simulink model "IEEE30_case"  (R2024b)
settings: Solver=FixedStepAuto  StartTime=0  StopTime=5  FixedStep=1e-7  RelTol=1e-3
values from neighbouring files (symbols this model uses):
  GFL_DFIG_7_C_bus = 0.08    [IEEE30_case_parameters.m]
  GFL_DFIG_7_D_mutual = 2.500000e+3    (= 2500)    [IEEE30_case_parameters.m]
  GFL_DFIG_7_f0 = 60    [IEEE30_case_parameters.m]
  GFL_DFIG_7_gPLLi = 3200    [IEEE30_case_parameters.m]
  GFL_DFIG_7_gPLLp = 650    [IEEE30_case_parameters.m]
  GFL_DFIG_7_H_WT = 0.4    [IEEE30_case_parameters.m]
  GFL_DFIG_7_Hg = 0.8    [IEEE30_case_parameters.m]
  GFL_DFIG_7_Igq_ref = 0    [IEEE30_case_parameters.m]
  GFL_DFIG_7_Ird_ref = 704.45696    [IEEE30_case_parameters.m]
  GFL_DFIG_7_KI_V = -300000    [IEEE30_case_parameters.m]
  GFL_DFIG_7_KP_V = -1000    [IEEE30_case_parameters.m]
  GFL_DFIG_7_Ksh = 1.254300e+4    (= 12543)    [IEEE30_case_parameters.m]
  GFL_DFIG_7_Lg = 0.000483    [IEEE30_case_parameters.m]
  GFL_DFIG_7_Lm_pu = 4    [IEEE30_case_parameters.m]
  GFL_DFIG_7_N = 100    [IEEE30_case_parameters.m]
  GFL_DFIG_7_p = 2    [IEEE30_case_parameters.m]
  GFL_DFIG_7_Pitch = 0    [IEEE30_case_parameters.m]
  GFL_DFIG_7_R = 44    [IEEE30_case_parameters.m]
  GFL_DFIG_7_Rg = 2.000000e-5    (= 2e-05)    [IEEE30_case_parameters.m]
  GFL_DFIG_7_rho = 1.225    [IEEE30_case_parameters.m]
  GFL_DFIG_7_rPLLi = 4500    [IEEE30_case_parameters.m]
  GFL_DFIG_7_rPLLp = 620    [IEEE30_case_parameters.m]
  GFL_DFIG_7_Rs_pu = 0.011    [IEEE30_case_parameters.m]
  GFL_DFIG_7_Sbase = 2.000000e+6    (= 2000000)    [IEEE30_case_parameters.m]
  GFL_DFIG_7_ugq_ref = 0    [IEEE30_case_parameters.m]
  GFL_DFIG_7_usd_ref = 0    [IEEE30_case_parameters.m]
  GFL_DFIG_7_Vbase = 690    [IEEE30_case_parameters.m]
  GFL_DFIG_7_Vdc_ref = 1200    [IEEE30_case_parameters.m]
  GFL_DFIG_7_wind = 12    [IEEE30_case_parameters.m]
  GFL_DFIG_7_wm_ref = 518.184209    [IEEE30_case_parameters.m]
  SG_D_13_D = 0.01056    [IEEE30_case_parameters.m]
  SG_D_13_EnableSaturation = 0    [IEEE30_case_parameters.m]
  SG_D_13_f0 = 60    [IEEE30_case_parameters.m]
  SG_D_13_H = 7.5    [IEEE30_case_parameters.m]
  SG_D_13_K_A = 20    [IEEE30_case_parameters.m]
  SG_D_13_K_E = 1.000000e+1    (= 10)    [IEEE30_case_parameters.m]
  SG_D_13_K_F = 2.363    [IEEE30_case_parameters.m]
  SG_D_13_K_s = 0.5    [IEEE30_case_parameters.m]
  SG_D_13_R_a = 0.001088    [IEEE30_case_parameters.m]
  SG_D_13_S_A = 1    [IEEE30_case_parameters.m]
  SG_D_13_S_B = 0.103    [IEEE30_case_parameters.m]
  SG_D_13_S_N = 10.659857    [IEEE30_case_parameters.m]
  SG_D_13_SpeedPara = 200    [IEEE30_case_parameters.m]
  SG_D_13_T_0 = 0.370163    [IEEE30_case_parameters.m]
  SG_D_13_T_1 = 0.3    [IEEE30_case_parameters.m]
  SG_D_13_T_2 = 0.05    [IEEE30_case_parameters.m]
  SG_D_13_T_3 = 0.02    [IEEE30_case_parameters.m]
  SG_D_13_T_4 = 0.005    [IEEE30_case_parameters.m]
  SG_D_13_T_A = 0.02    [IEEE30_case_parameters.m]
  SG_D_13_T_dd = 8.000000e+0    (= 8)    [IEEE30_case_parameters.m]
  SG_D_13_T_ddd = 0.04    [IEEE30_case_parameters.m]
  SG_D_13_T_E = 0.314    [IEEE30_case_parameters.m]
  SG_D_13_T_F = 0.35    [IEEE30_case_parameters.m]
  SG_D_13_T_qd = 0.8    [IEEE30_case_parameters.m]
  SG_D_13_T_qdd = 0.02    [IEEE30_case_parameters.m]
  SG_D_13_T_speed = 0.1    [IEEE30_case_parameters.m]
  SG_D_13_T_w = 0.5    [IEEE30_case_parameters.m]
  SG_D_13_V_ref = 1.696619    [IEEE30_case_parameters.m]
  SG_D_13_w_ref = 376.991118    [IEEE30_case_parameters.m]
  SG_D_13_x_d = 1.9    [IEEE30_case_parameters.m]
  SG_D_13_x_dd = 0.302    [IEEE30_case_parameters.m]
  SG_D_13_x_ddd = 0.204    [IEEE30_case_parameters.m]
  SG_D_13_x_l = 0.05    [IEEE30_case_parameters.m]
  SG_D_13_x_q = 1.3    [IEEE30_case_parameters.m]
  SG_D_13_x_qd = 0.5    [IEEE30_case_parameters.m]
  SG_D_13_x_qdd = 0.3    [IEEE30_case_parameters.m]
  SG_D_1_D = 0.01056    [IEEE30_case_parameters.m]
  SG_D_1_EnableSaturation = 0    [IEEE30_case_parameters.m]
  SG_D_1_f0 = 60    [IEEE30_case_parameters.m]
  SG_D_1_H = 7.5    [IEEE30_case_parameters.m]
  SG_D_1_K_A = 20    [IEEE30_case_parameters.m]
  SG_D_1_K_E = 1.000000e+1    (= 10)    [IEEE30_case_parameters.m]
  SG_D_1_K_F = 2.363    [IEEE30_case_parameters.m]
  SG_D_1_K_s = 0.5    [IEEE30_case_parameters.m]
  SG_D_1_R_a = 0.001088    [IEEE30_case_parameters.m]
  SG_D_1_S_A = 1    [IEEE30_case_parameters.m]
  SG_D_1_S_B = 0.103    [IEEE30_case_parameters.m]
  SG_D_1_S_N = 10.659857    [IEEE30_case_parameters.m]
  SG_D_1_SpeedPara = 200    [IEEE30_case_parameters.m]
  SG_D_1_T_0 = 0.259812    [IEEE30_case_parameters.m]
  SG_D_1_T_1 = 0.3    [IEEE30_case_parameters.m]
  SG_D_1_T_2 = 0.05    [IEEE30_case_parameters.m]
  SG_D_1_T_3 = 0.02    [IEEE30_case_parameters.m]
  SG_D_1_T_4 = 0.005    [IEEE30_case_parameters.m]
  SG_D_1_T_A = 0.02    [IEEE30_case_parameters.m]
  SG_D_1_T_dd = 8.000000e+0    (= 8)    [IEEE30_case_parameters.m]
  SG_D_1_T_ddd = 0.04    [IEEE30_case_parameters.m]
  SG_D_1_T_E = 0.314    [IEEE30_case_parameters.m]
  SG_D_1_T_F = 0.35    [IEEE30_case_parameters.m]
  SG_D_1_T_qd = 0.8    [IEEE30_case_parameters.m]
  SG_D_1_T_qdd = 0.02    [IEEE30_case_parameters.m]
  SG_D_1_T_speed = 0.1    [IEEE30_case_parameters.m]
  SG_D_1_T_w = 0.5    [IEEE30_case_parameters.m]
  SG_D_1_V_ref = 1.544107    [IEEE30_case_parameters.m]
  SG_D_1_w_ref = 376.991118    [IEEE30_case_parameters.m]
  SG_D_1_x_d = 1.9    [IEEE30_case_parameters.m]
  SG_D_1_x_dd = 0.302    [IEEE30_case_parameters.m]
  SG_D_1_x_ddd = 0.204    [IEEE30_case_parameters.m]
  SG_D_1_x_l = 0.05    [IEEE30_case_parameters.m]
  SG_D_1_x_q = 1.3    [IEEE30_case_parameters.m]
  SG_D_1_x_qd = 0.5    [IEEE30_case_parameters.m]
  SG_D_1_x_qdd = 0.3    [IEEE30_case_parameters.m]
  SG_D_22_D = 0.01056    [IEEE30_case_parameters.m]
  SG_D_22_EnableSaturation = 0    [IEEE30_case_parameters.m]
  SG_D_22_f0 = 60    [IEEE30_case_parameters.m]
  SG_D_22_H = 7.5    [IEEE30_case_parameters.m]
  SG_D_22_K_A = 20    [IEEE30_case_parameters.m]
  SG_D_22_K_E = 1.000000e+1    (= 10)    [IEEE30_case_parameters.m]
  SG_D_22_K_F = 2.363    [IEEE30_case_parameters.m]
  SG_D_22_K_s = 0.5    [IEEE30_case_parameters.m]
  SG_D_22_R_a = 0.001088    [IEEE30_case_parameters.m]
  SG_D_22_S_A = 1    [IEEE30_case_parameters.m]
  SG_D_22_S_B = 0.103    [IEEE30_case_parameters.m]
  SG_D_22_S_N = 10.659857    [IEEE30_case_parameters.m]
  SG_D_22_SpeedPara = 200    [IEEE30_case_parameters.m]
  SG_D_22_T_0 = 0.216121    [IEEE30_case_parameters.m]
  SG_D_22_T_1 = 0.3    [IEEE30_case_parameters.m]
  SG_D_22_T_2 = 0.05    [IEEE30_case_parameters.m]
  SG_D_22_T_3 = 0.02    [IEEE30_case_parameters.m]
  SG_D_22_T_4 = 0.005    [IEEE30_case_parameters.m]
  ... (+126 more)
(part 11 of 27)

== system IEEE30_case/AC_1/iq_bus_12_block ==
  note: iq_bus_12 in IEEE30_case
      | $\mathrm{iq}_{\mathrm{line},4,12}-\mathrm{iq}_{\mathrm{load},12}-\mathrm{iq}_{\mathrm{line},12,13}-\mathrm{iq}_{\mathrm{line},12,14}-\mathrm{iq}_{\mathrm{line},12,15}-\mathrm{iq}_{\mathrm{line},12,16}$
      | Automatically generated on 2025-11-01 18:42:55 .
  State_iq_load_12_bc973 : Inport
  State_iq_line_4_12_d3882 : Inport  Port=2
  State_iq_line_12_13_64934 : Inport  Port=3
  State_iq_line_12_14_05407 : Inport  Port=4
  State_iq_line_12_15_032f0 : Inport  Port=5
  State_iq_line_12_16_bc787 : Inport  Port=6
  Add_841f8 : Sum
  Constant_-1_4865d : Constant  Value=-1
  Product_64089 : Product
  Subtract_44be1 : Sum  Inputs=+-
  Subtract_8e198 : Sum  Inputs=+-
  Subtract_b2fb8 : Sum  Inputs=+-
  Subtract_d73aa : Sum  Inputs=+-
  Blockout_iq_bus_12_94dfd : Outport
  wires:
  State_iq_line_4_12_d3882/1 -> Add_841f8/2
  Constant_-1_4865d/1 -> Product_64089/1
  Product_64089/1 -> Add_841f8/1
  State_iq_load_12_bc973/1 -> Product_64089/2
  State_iq_line_12_14_05407/1 -> Subtract_44be1/2
  Subtract_8e198/1 -> Subtract_d73aa/1
  Add_841f8/1 -> Subtract_b2fb8/1
  Subtract_b2fb8/1 -> Subtract_44be1/1
  State_iq_line_12_13_64934/1 -> Subtract_b2fb8/2
  Subtract_44be1/1 -> Subtract_8e198/1
  State_iq_line_12_15_032f0/1 -> Subtract_8e198/2
  State_iq_line_12_16_bc787/1 -> Subtract_d73aa/2
  Subtract_d73aa/1 -> Blockout_iq_bus_12_94dfd/1

== system IEEE30_case/AC_1/iq_bus_13_block ==
  note: iq_bus_13 in IEEE30_case
      | $\mathrm{iq}_{\mathrm{SG},D,13}+\mathrm{iq}_{\mathrm{line},12,13}$
      | Automatically generated on 2025-11-01 18:42:58 .
  Input_iq_SG_D_13_41b6f : Inport
  State_iq_line_12_13_2e588 : Inport  Port=2
  Add_10a27 : Sum
  Blockout_iq_bus_13_72f64 : Outport
  wires:
  Input_iq_SG_D_13_41b6f/1 -> Add_10a27/1
  State_iq_line_12_13_2e588/1 -> Add_10a27/2
  Add_10a27/1 -> Blockout_iq_bus_13_72f64/1

== system IEEE30_case/AC_1/iq_bus_14_block ==
  note: iq_bus_14 in IEEE30_case
      | $\mathrm{iq}_{\mathrm{line},12,14}-\mathrm{iq}_{\mathrm{load},14}-\mathrm{iq}_{\mathrm{line},14,15}$
      | Automatically generated on 2025-11-01 18:42:59 .
  State_iq_load_14_72e79 : Inport
  State_iq_line_12_14_c9961 : Inport  Port=2
  State_iq_line_14_15_62994 : Inport  Port=3
  Add_1995a : Sum
  Constant_-1_aea63 : Constant  Value=-1
  Product_4bd77 : Product
  Subtract_3c8e1 : Sum  Inputs=+-
  Blockout_iq_bus_14_40877 : Outport
  wires:
  State_iq_line_14_15_62994/1 -> Subtract_3c8e1/2
  State_iq_line_12_14_c9961/1 -> Add_1995a/2
  Product_4bd77/1 -> Add_1995a/1
  Constant_-1_aea63/1 -> Product_4bd77/1
  State_iq_load_14_72e79/1 -> Product_4bd77/2
  Add_1995a/1 -> Subtract_3c8e1/1
  Subtract_3c8e1/1 -> Blockout_iq_bus_14_40877/1

== system IEEE30_case/AC_1/iq_bus_15_block ==
  note: iq_bus_15 in IEEE30_case
      | $\mathrm{iq}_{\mathrm{line},12,15}-\mathrm{iq}_{\mathrm{load},15}+\mathrm{iq}_{\mathrm{line},14,15}-\mathrm{iq}_{\mathrm{line},15,18}-\mathrm{iq}_{\mathrm{line},15,23}$
      | Automatically generated on 2025-11-01 18:43:01 .
  State_iq_load_15_d1891 : Inport
  State_iq_line_12_15_d11d7 : Inport  Port=2
  State_iq_line_14_15_cd3f2 : Inport  Port=3
  State_iq_line_15_18_a2738 : Inport  Port=4
  State_iq_line_15_23_dd72a : Inport  Port=5
  Add_86658 : Sum
  Add_f7d0d : Sum
  Constant_-1_2c9e4 : Constant  Value=-1
  Product_847ef : Product
  Subtract_29d9d : Sum  Inputs=+-
  Subtract_4ac4f : Sum  Inputs=+-
  Blockout_iq_bus_15_ccbd2 : Outport
  wires:
  State_iq_line_14_15_cd3f2/1 -> Add_f7d0d/2
  Subtract_4ac4f/1 -> Subtract_29d9d/1
  State_iq_line_12_15_d11d7/1 -> Add_86658/2
  Constant_-1_2c9e4/1 -> Product_847ef/1
  Product_847ef/1 -> Add_86658/1
  State_iq_load_15_d1891/1 -> Product_847ef/2
  State_iq_line_15_18_a2738/1 -> Subtract_4ac4f/2
  Add_86658/1 -> Add_f7d0d/1
  Add_f7d0d/1 -> Subtract_4ac4f/1
  State_iq_line_15_23_dd72a/1 -> Subtract_29d9d/2
  Subtract_29d9d/1 -> Blockout_iq_bus_15_ccbd2/1

== system IEEE30_case/AC_1/iq_bus_16_block ==
  note: iq_bus_16 in IEEE30_case
      | $\mathrm{iq}_{\mathrm{line},12,16}-\mathrm{iq}_{\mathrm{load},16}-\mathrm{iq}_{\mathrm{line},16,17}$
      | Automatically generated on 2025-11-01 18:43:03 .
  State_iq_load_16_aacc5 : Inport
  State_iq_line_12_16_8d22f : Inport  Port=2
  State_iq_line_16_17_2d89b : Inport  Port=3
  Add_8c6a6 : Sum
  Constant_-1_7911e : Constant  Value=-1
  Product_fbab2 : Product
  Subtract_cf134 : Sum  Inputs=+-
  Blockout_iq_bus_16_0845b : Outport
  wires:
  Product_fbab2/1 -> Add_8c6a6/1
  Constant_-1_7911e/1 -> Product_fbab2/1
  State_iq_load_16_aacc5/1 -> Product_fbab2/2
  State_iq_line_16_17_2d89b/1 -> Subtract_cf134/2
  Add_8c6a6/1 -> Subtract_cf134/1
  State_iq_line_12_16_8d22f/1 -> Add_8c6a6/2
  Subtract_cf134/1 -> Blockout_iq_bus_16_0845b/1

== system IEEE30_case/AC_1/iq_bus_17_block ==
  note: iq_bus_17 in IEEE30_case
      | $\mathrm{iq}_{\mathrm{line},10,17}-\mathrm{iq}_{\mathrm{load},17}+\mathrm{iq}_{\mathrm{line},16,17}$
      | Automatically generated on 2025-11-01 18:43:05 .
  State_iq_load_17_c996c : Inport
  State_iq_line_10_17_8adde : Inport  Port=2
  State_iq_line_16_17_d8ac8 : Inport  Port=3
  Add_26423 : Sum
  Add_c9bbe : Sum
  Constant_-1_1ae42 : Constant  Value=-1
  Product_876e2 : Product
  Blockout_iq_bus_17_f1a33 : Outport
  wires:
  Add_c9bbe/1 -> Blockout_iq_bus_17_f1a33/1
  Constant_-1_1ae42/1 -> Product_876e2/1
  State_iq_load_17_c996c/1 -> Product_876e2/2
  Product_876e2/1 -> Add_26423/1
  State_iq_line_16_17_d8ac8/1 -> Add_c9bbe/2
  Add_26423/1 -> Add_c9bbe/1
  State_iq_line_10_17_8adde/1 -> Add_26423/2

== system IEEE30_case/AC_1/iq_bus_18_block ==
  note: iq_bus_18 in IEEE30_case
      | $\mathrm{iq}_{\mathrm{line},15,18}-\mathrm{iq}_{\mathrm{load},18}-\mathrm{iq}_{\mathrm{line},18,19}$
      | Automatically generated on 2025-11-01 18:43:06 .
  State_iq_load_18_b73eb : Inport
  State_iq_line_15_18_3f1e8 : Inport  Port=2
  State_iq_line_18_19_1de76 : Inport  Port=3
  Add_094f5 : Sum
  Constant_-1_fe84d : Constant  Value=-1
  Product_a729b : Product
  Subtract_f2aa7 : Sum  Inputs=+-
  Blockout_iq_bus_18_b4916 : Outport
  wires:
  Subtract_f2aa7/1 -> Blockout_iq_bus_18_b4916/1
  Product_a729b/1 -> Add_094f5/1
  Constant_-1_fe84d/1 -> Product_a729b/1
  State_iq_line_15_18_3f1e8/1 -> Add_094f5/2
  State_iq_load_18_b73eb/1 -> Product_a729b/2
  Add_094f5/1 -> Subtract_f2aa7/1
  State_iq_line_18_19_1de76/1 -> Subtract_f2aa7/2

== system IEEE30_case/AC_1/iq_bus_19_block ==
  note: iq_bus_19 in IEEE30_case
      | $\mathrm{iq}_{\mathrm{line},18,19}-\mathrm{iq}_{\mathrm{load},19}-\mathrm{iq}_{\mathrm{line},19,20}$
      | Automatically generated on 2025-11-01 18:43:08 .
  State_iq_load_19_c9423 : Inport
  State_iq_line_18_19_b0a61 : Inport  Port=2
  State_iq_line_19_20_3626a : Inport  Port=3
  Add_da601 : Sum
  Constant_-1_3887f : Constant  Value=-1
  Product_3a158 : Product
  Subtract_a6f15 : Sum  Inputs=+-
  Blockout_iq_bus_19_07988 : Outport
  wires:
  State_iq_line_18_19_b0a61/1 -> Add_da601/2
  Product_3a158/1 -> Add_da601/1
  Constant_-1_3887f/1 -> Product_3a158/1
  State_iq_load_19_c9423/1 -> Product_3a158/2
  Add_da601/1 -> Subtract_a6f15/1
  State_iq_line_19_20_3626a/1 -> Subtract_a6f15/2
  Subtract_a6f15/1 -> Blockout_iq_bus_19_07988/1

== system IEEE30_case/AC_1/iq_bus_1_block ==
  note: iq_bus_1 in IEEE30_case
      | $\mathrm{iq}_{\mathrm{SG},D,1}-\mathrm{iq}_{\mathrm{line},1,2}-\mathrm{iq}_{\mathrm{line},1,3}$
      | Automatically generated on 2025-11-01 18:42:34 .
  Input_iq_SG_D_1_636be : Inport
  State_iq_line_1_2_426df : Inport  Port=2
  State_iq_line_1_3_a1a02 : Inport  Port=3
  Subtract_baca8 : Sum  Inputs=+-
  Subtract_effd5 : Sum  Inputs=+-
  Blockout_iq_bus_1_c22d8 : Outport
  wires:
  Subtract_baca8/1 -> Blockout_iq_bus_1_c22d8/1
  Input_iq_SG_D_1_636be/1 -> Subtract_effd5/1
  State_iq_line_1_3_a1a02/1 -> Subtract_baca8/2
  State_iq_line_1_2_426df/1 -> Subtract_effd5/2
  Subtract_effd5/1 -> Subtract_baca8/1

== system IEEE30_case/AC_1/iq_bus_20_block ==
  note: iq_bus_20 in IEEE30_case
      | $\mathrm{iq}_{\mathrm{line},10,20}-\mathrm{iq}_{\mathrm{load},20}+\mathrm{iq}_{\mathrm{line},19,20}$
      | Automatically generated on 2025-11-01 18:43:10 .
  State_iq_load_20_1f6b7 : Inport
  State_iq_line_10_20_d570b : Inport  Port=2
  State_iq_line_19_20_435ec : Inport  Port=3
  Add_2092f : Sum
  Add_2fcde : Sum
  Constant_-1_9ffd8 : Constant  Value=-1
  Product_27044 : Product
  Blockout_iq_bus_20_faa95 : Outport
  wires:
  Add_2092f/1 -> Add_2fcde/1
  Product_27044/1 -> Add_2092f/1
  Constant_-1_9ffd8/1 -> Product_27044/1
  State_iq_load_20_1f6b7/1 -> Product_27044/2
  Add_2fcde/1 -> Blockout_iq_bus_20_faa95/1
  State_iq_line_19_20_435ec/1 -> Add_2fcde/2
  State_iq_line_10_20_d570b/1 -> Add_2092f/2

== system IEEE30_case/AC_1/iq_bus_21_block ==
  note: iq_bus_21 in IEEE30_case
      | $\mathrm{iq}_{\mathrm{line},10,21}-\mathrm{iq}_{\mathrm{load},21}-\mathrm{iq}_{\mathrm{line},21,22}$
      | Automatically generated on 2025-11-01 18:43:11 .
  State_iq_load_21_44508 : Inport
  State_iq_line_10_21_86c36 : Inport  Port=2
  State_iq_line_21_22_832b6 : Inport  Port=3
  Add_22f1e : Sum
  Constant_-1_58c82 : Constant  Value=-1
  Product_c246b : Product
  Subtract_625b5 : Sum  Inputs=+-
  Blockout_iq_bus_21_51471 : Outport
  wires:
  State_iq_line_21_22_832b6/1 -> Subtract_625b5/2
  State_iq_line_10_21_86c36/1 -> Add_22f1e/2
  Constant_-1_58c82/1 -> Product_c246b/1
  State_iq_load_21_44508/1 -> Product_c246b/2
  Product_c246b/1 -> Add_22f1e/1
  Add_22f1e/1 -> Subtract_625b5/1
  Subtract_625b5/1 -> Blockout_iq_bus_21_51471/1

== system IEEE30_case/AC_1/iq_bus_22_block ==
  note: iq_bus_22 in IEEE30_case
      | $\mathrm{iq}_{\mathrm{SG},D,22}+\mathrm{iq}_{\mathrm{line},10,22}+\mathrm{iq}_{\mathrm{line},21,22}-\mathrm{iq}_{\mathrm{line},22,24}$
      | Automatically generated on 2025-11-01 18:43:14 .
  Input_iq_SG_D_22_7afaf : Inport
  State_iq_line_10_22_172f8 : Inport  Port=2
  State_iq_line_21_22_a7d32 : Inport  Port=3
  State_iq_line_22_24_573df : Inport  Port=4
  Add_60857 : Sum
  Add_ff722 : Sum
  Subtract_94456 : Sum  Inputs=+-
  Blockout_iq_bus_22_6516e : Outport
  wires:
  Subtract_94456/1 -> Blockout_iq_bus_22_6516e/1
  Add_ff722/1 -> Add_60857/1
  Input_iq_SG_D_22_7afaf/1 -> Add_ff722/1
  State_iq_line_10_22_172f8/1 -> Add_ff722/2
  Add_60857/1 -> Subtract_94456/1
  State_iq_line_21_22_a7d32/1 -> Add_60857/2
  State_iq_line_22_24_573df/1 -> Subtract_94456/2

== system IEEE30_case/AC_1/iq_bus_23_block ==
  note: iq_bus_23 in IEEE30_case
      | $\mathrm{iq}_{\mathrm{SG},D,23}-\mathrm{iq}_{\mathrm{load},23}+\mathrm{iq}_{\mathrm{line},15,23}-\mathrm{iq}_{\mathrm{line},23,24}$
      | Automatically generated on 2025-11-01 18:43:17 .
  Input_iq_SG_D_23_15e34 : Inport
  State_iq_load_23_12e45 : Inport  Port=2
  State_iq_line_15_23_fc0a9 : Inport  Port=3
  State_iq_line_23_24_17ece : Inport  Port=4
  Add_e4154 : Sum
  Subtract_5918e : Sum  Inputs=+-
  Subtract_8e4ad : Sum  Inputs=+-
  Blockout_iq_bus_23_896ad : Outport
  wires:
  Subtract_8e4ad/1 -> Add_e4154/1
  Input_iq_SG_D_23_15e34/1 -> Subtract_8e4ad/1
  State_iq_load_23_12e45/1 -> Subtract_8e4ad/2
  State_iq_line_23_24_17ece/1 -> Subtract_5918e/2
  Add_e4154/1 -> Subtract_5918e/1
  State_iq_line_15_23_fc0a9/1 -> Add_e4154/2
  Subtract_5918e/1 -> Blockout_iq_bus_23_896ad/1

== system IEEE30_case/AC_1/iq_bus_24_block ==
  note: iq_bus_24 in IEEE30_case
      | $\mathrm{iq}_{\mathrm{line},22,24}-\mathrm{iq}_{\mathrm{load},24}+\mathrm{iq}_{\mathrm{line},23,24}-\mathrm{iq}_{\mathrm{line},24,25}$
      | Automatically generated on 2025-11-01 18:43:19 .
  State_iq_load_24_fdcb6 : Inport
  State_iq_line_22_24_76281 : Inport  Port=2
  State_iq_line_23_24_946d1 : Inport  Port=3
  State_iq_line_24_25_99c0f : Inport  Port=4
  Add_5c6aa : Sum
  Add_67e83 : Sum
  Constant_-1_ac1a7 : Constant  Value=-1
  Product_7a246 : Product
  Subtract_26d4f : Sum  Inputs=+-
  Blockout_iq_bus_24_a8f54 : Outport
  wires:
  Constant_-1_ac1a7/1 -> Product_7a246/1
  Product_7a246/1 -> Add_5c6aa/1
  Add_67e83/1 -> Subtract_26d4f/1
  Add_5c6aa/1 -> Add_67e83/1
  State_iq_load_24_fdcb6/1 -> Product_7a246/2
  State_iq_line_22_24_76281/1 -> Add_5c6aa/2
  State_iq_line_24_25_99c0f/1 -> Subtract_26d4f/2
  State_iq_line_23_24_946d1/1 -> Add_67e83/2
  Subtract_26d4f/1 -> Blockout_iq_bus_24_a8f54/1

== system IEEE30_case/AC_1/iq_bus_25_block ==
  note: iq_bus_25 in IEEE30_case
      | $\mathrm{iq}_{\mathrm{line},24,25}-\mathrm{iq}_{\mathrm{line},25,26}-\mathrm{iq}_{\mathrm{line},25,27}$
      | Automatically generated on 2025-11-01 18:43:21 .
  State_iq_line_24_25_0047e : Inport
  State_iq_line_25_26_b28ea : Inport  Port=2
  State_iq_line_25_27_6cee1 : Inport  Port=3
  Subtract_623d2 : Sum  Inputs=+-
  Subtract_b39cd : Sum  Inputs=+-
  Blockout_iq_bus_25_a2b76 : Outport
  wires:
  Subtract_b39cd/1 -> Blockout_iq_bus_25_a2b76/1
  State_iq_line_24_25_0047e/1 -> Subtract_623d2/1
  State_iq_line_25_26_b28ea/1 -> Subtract_623d2/2
  State_iq_line_25_27_6cee1/1 -> Subtract_b39cd/2
  Subtract_623d2/1 -> Subtract_b39cd/1

== system IEEE30_case/AC_1/iq_bus_26_block ==
  note: iq_bus_26 in IEEE30_case
      | $\mathrm{iq}_{\mathrm{line},25,26}-\mathrm{iq}_{\mathrm{load},26}$
      | Automatically generated on 2025-11-01 18:43:22 .
  State_iq_load_26_ac2a5 : Inport
  State_iq_line_25_26_3a876 : Inport  Port=2
  Add_463e9 : Sum
  Constant_-1_82269 : Constant  Value=-1
  Product_c91b9 : Product
  Blockout_iq_bus_26_d1a08 : Outport
  wires:
  Constant_-1_82269/1 -> Product_c91b9/1
  State_iq_line_25_26_3a876/1 -> Add_463e9/2
  Product_c91b9/1 -> Add_463e9/1
  State_iq_load_26_ac2a5/1 -> Product_c91b9/2
  Add_463e9/1 -> Blockout_iq_bus_26_d1a08/1

== system IEEE30_case/AC_1/iq_bus_27_block ==
  note: iq_bus_27 in IEEE30_case
      | $\mathrm{iq}_{\mathrm{SG},D,27}+\mathrm{iq}_{\mathrm{line},25,27}-\mathrm{iq}_{\mathrm{line},27,29}-\mathrm{iq}_{\mathrm{line},27,30}+\mathrm{iq}_{\mathrm{line},28,27}$
      | Automatically generated on 2025-11-01 18:43:25 .
  Input_iq_SG_D_27_5f248 : Inport
  State_iq_line_25_27_786f4 : Inport  Port=2
  State_iq_line_27_29_e7090 : Inport  Port=3
  State_iq_line_27_30_e8aeb : Inport  Port=4
  State_iq_line_28_27_c8698 : Inport  Port=5
  Add_88ff4 : Sum
  Add_a91b2 : Sum
  Subtract_49574 : Sum  Inputs=+-
  Subtract_f659e : Sum  Inputs=+-
  Blockout_iq_bus_27_6c5f3 : Outport
  wires:
  Subtract_f659e/1 -> Add_88ff4/1
  Input_iq_SG_D_27_5f248/1 -> Add_a91b2/1
  Add_a91b2/1 -> Subtract_49574/1
  Subtract_49574/1 -> Subtract_f659e/1
  State_iq_line_25_27_786f4/1 -> Add_a91b2/2
  State_iq_line_27_29_e7090/1 -> Subtract_49574/2
  State_iq_line_28_27_c8698/1 -> Add_88ff4/2
  State_iq_line_27_30_e8aeb/1 -> Subtract_f659e/2
  Add_88ff4/1 -> Blockout_iq_bus_27_6c5f3/1

== system IEEE30_case/AC_1/iq_bus_28_block ==
  note: iq_bus_28 in IEEE30_case
      | $\mathrm{iq}_{\mathrm{line},6,28}+\mathrm{iq}_{\mathrm{line},8,28}-\mathrm{iq}_{\mathrm{line},28,27}$
      | Automatically generated on 2025-11-01 18:43:27 .
  State_iq_line_6_28_9fc56 : Inport
  State_iq_line_8_28_5df2a : Inport  Port=2
  State_iq_line_28_27_5cab2 : Inport  Port=3
  Add_68cf3 : Sum
  Subtract_c2c34 : Sum  Inputs=+-
  Blockout_iq_bus_28_fc1de : Outport
  wires:
  Subtract_c2c34/1 -> Blockout_iq_bus_28_fc1de/1
  State_iq_line_6_28_9fc56/1 -> Add_68cf3/1
  State_iq_line_8_28_5df2a/1 -> Add_68cf3/2
  Add_68cf3/1 -> Subtract_c2c34/1
  State_iq_line_28_27_5cab2/1 -> Subtract_c2c34/2

== system IEEE30_case/AC_1/iq_bus_29_block ==
  note: iq_bus_29 in IEEE30_case
      | $\mathrm{iq}_{\mathrm{line},27,29}-\mathrm{iq}_{\mathrm{load},29}-\mathrm{iq}_{\mathrm{line},29,30}$
      | Automatically generated on 2025-11-01 18:43:28 .
  State_iq_load_29_82b4e : Inport
  State_iq_line_27_29_eb40a : Inport  Port=2
  State_iq_line_29_30_aaab3 : Inport  Port=3
  Add_05210 : Sum
  Constant_-1_1f122 : Constant  Value=-1
  Product_41592 : Product
  Subtract_864dd : Sum  Inputs=+-
  Blockout_iq_bus_29_54fcd : Outport
  wires:
  Subtract_864dd/1 -> Blockout_iq_bus_29_54fcd/1
  Product_41592/1 -> Add_05210/1
  Constant_-1_1f122/1 -> Product_41592/1
  State_iq_load_29_82b4e/1 -> Product_41592/2
  State_iq_line_27_29_eb40a/1 -> Add_05210/2
  Add_05210/1 -> Subtract_864dd/1
  State_iq_line_29_30_aaab3/1 -> Subtract_864dd/2

== system IEEE30_case/AC_1/iq_bus_2_block ==
  note: iq_bus_2 in IEEE30_case
      | $\mathrm{iq}_{\mathrm{SG},D,2}-\mathrm{iq}_{\mathrm{load},2}+\mathrm{iq}_{\mathrm{line},1,2}-\mathrm{iq}_{\mathrm{line},2,4}-\mathrm{iq}_{\mathrm{line},2,5}-\mathrm{iq}_{\mathrm{line},2,6}$
      | Automatically generated on 2025-11-01 18:42:36 .
  Input_iq_SG_D_2_3deae : Inport
  State_iq_load_2_becb6 : Inport  Port=2
  State_iq_line_1_2_22297 : Inport  Port=3
  State_iq_line_2_4_c1409 : Inport  Port=4
  State_iq_line_2_5_9d19f : Inport  Port=5
  State_iq_line_2_6_42b8c : Inport  Port=6
  Add_32615 : Sum
  Subtract_354fb : Sum  Inputs=+-
  Subtract_3c630 : Sum  Inputs=+-
  Subtract_b2643 : Sum  Inputs=+-
  Subtract_bac10 : Sum  Inputs=+-
  Blockout_iq_bus_2_bb89e : Outport
  wires:
  State_iq_line_1_2_22297/1 -> Add_32615/2
  Input_iq_SG_D_2_3deae/1 -> Subtract_b2643/1
  Subtract_b2643/1 -> Add_32615/1
  State_iq_load_2_becb6/1 -> Subtract_b2643/2
  State_iq_line_2_5_9d19f/1 -> Subtract_354fb/2
  State_iq_line_2_4_c1409/1 -> Subtract_bac10/2
  Add_32615/1 -> Subtract_bac10/1
  Subtract_bac10/1 -> Subtract_354fb/1
  Subtract_354fb/1 -> Subtract_3c630/1
  State_iq_line_2_6_42b8c/1 -> Subtract_3c630/2
  Subtract_3c630/1 -> Blockout_iq_bus_2_bb89e/1

== system IEEE30_case/AC_1/iq_bus_30_block ==
  note: iq_bus_30 in IEEE30_case
      | $\mathrm{iq}_{\mathrm{line},27,30}-\mathrm{iq}_{\mathrm{load},30}+\mathrm{iq}_{\mathrm{line},29,30}$
      | Automatically generated on 2025-11-01 18:43:30 .
  State_iq_load_30_e4c4c : Inport
  State_iq_line_27_30_c3531 : Inport  Port=2
  State_iq_line_29_30_a165e : Inport  Port=3
  Add_2918f : Sum
  Add_b8be3 : Sum
  Constant_-1_8c75b : Constant  Value=-1
  Product_583d8 : Product
  Blockout_iq_bus_30_f5578 : Outport
  wires:
  State_iq_line_29_30_a165e/1 -> Add_b8be3/2
  State_iq_line_27_30_c3531/1 -> Add_2918f/2
  Product_583d8/1 -> Add_2918f/1
  Constant_-1_8c75b/1 -> Product_583d8/1
  State_iq_load_30_e4c4c/1 -> Product_583d8/2
  Add_2918f/1 -> Add_b8be3/1
  Add_b8be3/1 -> Blockout_iq_bus_30_f5578/1

== system IEEE30_case/AC_1/iq_bus_3_block ==
  note: iq_bus_3 in IEEE30_case
      | $\mathrm{iq}_{\mathrm{line},1,3}-\mathrm{iq}_{\mathrm{load},3}-\mathrm{iq}_{\mathrm{line},3,4}$
      | Automatically generated on 2025-11-01 18:42:38 .
  State_iq_load_3_98680 : Inport
  State_iq_line_1_3_704f9 : Inport  Port=2
  State_iq_line_3_4_e67cb : Inport  Port=3
  Add_9cf2e : Sum
  Constant_-1_14019 : Constant  Value=-1
  Product_a35fa : Product
  Subtract_a74b4 : Sum  Inputs=+-
  Blockout_iq_bus_3_0811d : Outport
  wires:
  Product_a35fa/1 -> Add_9cf2e/1
  Constant_-1_14019/1 -> Product_a35fa/1
  State_iq_load_3_98680/1 -> Product_a35fa/2
  Add_9cf2e/1 -> Subtract_a74b4/1
  State_iq_line_1_3_704f9/1 -> Add_9cf2e/2
  State_iq_line_3_4_e67cb/1 -> Subtract_a74b4/2
  Subtract_a74b4/1 -> Blockout_iq_bus_3_0811d/1

== system IEEE30_case/AC_1/iq_bus_4_block ==
  note: iq_bus_4 in IEEE30_case
      | $\mathrm{iq}_{\mathrm{line},2,4}-\mathrm{iq}_{\mathrm{load},4}+\mathrm{iq}_{\mathrm{line},3,4}-\mathrm{iq}_{\mathrm{line},4,6}-\mathrm{iq}_{\mathrm{line},4,12}$
      | Automatically generated on 2025-11-01 18:42:40 .
  State_iq_load_4_0a7a4 : Inport
  State_iq_line_2_4_37eb2 : Inport  Port=2
  State_iq_line_3_4_5b109 : Inport  Port=3
  State_iq_line_4_6_d2f2a : Inport  Port=4
  State_iq_line_4_12_8cce3 : Inport  Port=5
  Add_5198b : Sum
  Add_8557f : Sum
  Constant_-1_cc943 : Constant  Value=-1
  Product_6109f : Product
  Subtract_850d4 : Sum  Inputs=+-
  Subtract_9ef8a : Sum  Inputs=+-
  Blockout_iq_bus_4_c8ef1 : Outport
  wires:
  Constant_-1_cc943/1 -> Product_6109f/1
  Product_6109f/1 -> Add_8557f/1
  State_iq_load_4_0a7a4/1 -> Product_6109f/2
  State_iq_line_2_4_37eb2/1 -> Add_8557f/2
  Add_8557f/1 -> Add_5198b/1
  State_iq_line_4_6_d2f2a/1 -> Subtract_850d4/2
  State_iq_line_3_4_5b109/1 -> Add_5198b/2
  Add_5198b/1 -> Subtract_850d4/1
  Subtract_850d4/1 -> Subtract_9ef8a/1
  State_iq_line_4_12_8cce3/1 -> Subtract_9ef8a/2
  Subtract_9ef8a/1 -> Blockout_iq_bus_4_c8ef1/1

== system IEEE30_case/AC_1/iq_bus_5_block ==
  note: iq_bus_5 in IEEE30_case
      | $\mathrm{iq}_{\mathrm{line},2,5}-\mathrm{iq}_{\mathrm{line},5,7}$
      | Automatically generated on 2025-11-01 18:42:41 .
  State_iq_line_2_5_98d2b : Inport
  State_iq_line_5_7_0b183 : Inport  Port=2
  Subtract_b6711 : Sum  Inputs=+-
  Blockout_iq_bus_5_aa6f8 : Outport
  wires:
  State_iq_line_5_7_0b183/1 -> Subtract_b6711/2
  State_iq_line_2_5_98d2b/1 -> Subtract_b6711/1
  Subtract_b6711/1 -> Blockout_iq_bus_5_aa6f8/1

== system IEEE30_case/AC_1/iq_bus_6_block ==
  note: iq_bus_6 in IEEE30_case
      | $\mathrm{iq}_{\mathrm{line},2,6}+\mathrm{iq}_{\mathrm{line},4,6}-\mathrm{iq}_{\mathrm{line},6,7}-\mathrm{iq}_{\mathrm{line},6,8}-\mathrm{iq}_{\mathrm{line},6,9}-\mathrm{iq}_{\mathrm{line},6,10}-\mathrm{iq}_{\mathrm{line},6,28}$
      | Automatically generated on 2025-11-01 18:42:44 .
  State_iq_line_2_6_0b501 : Inport
  State_iq_line_4_6_7829d : Inport  Port=2
  State_iq_line_6_7_5270c : Inport  Port=3
  State_iq_line_6_8_410de : Inport  Port=4
  State_iq_line_6_9_51dc2 : Inport  Port=5
  State_iq_line_6_10_0da9e : Inport  Port=6
  State_iq_line_6_28_c6c23 : Inport  Port=7
  Add_66cb7 : Sum
  Subtract_384c7 : Sum  Inputs=+-
  Subtract_3e05f : Sum  Inputs=+-
  Subtract_4ae4e : Sum  Inputs=+-
  Subtract_adbcc : Sum  Inputs=+-
  Subtract_b388f : Sum  Inputs=+-
  Blockout_iq_bus_6_4f954 : Outport
  wires:
  State_iq_line_2_6_0b501/1 -> Add_66cb7/1
  State_iq_line_4_6_7829d/1 -> Add_66cb7/2
  Add_66cb7/1 -> Subtract_3e05f/1
  Subtract_3e05f/1 -> Subtract_adbcc/1
  State_iq_line_6_8_410de/1 -> Subtract_adbcc/2
  State_iq_line_6_7_5270c/1 -> Subtract_3e05f/2
  Subtract_b388f/1 -> Subtract_4ae4e/1
  Subtract_adbcc/1 -> Subtract_384c7/1
  State_iq_line_6_9_51dc2/1 -> Subtract_384c7/2
  Subtract_384c7/1 -> Subtract_b388f/1
  State_iq_line_6_10_0da9e/1 -> Subtract_b388f/2
  State_iq_line_6_28_c6c23/1 -> Subtract_4ae4e/2
  Subtract_4ae4e/1 -> Blockout_iq_bus_6_4f954/1

== system IEEE30_case/AC_1/iq_bus_7_block ==
  note: iq_bus_7 in IEEE30_case
      | $\mathrm{iq}_{\mathrm{line},5,7}-\mathrm{iq}_{\mathrm{load},7}+\mathrm{iq}_{\mathrm{line},6,7}+\mathrm{iq}_{\mathrm{GFL},\mathrm{DFIG},7}$
      | Automatically generated on 2025-11-01 18:42:47 .
  Input_iq_GFL_DFIG_7_603eb : Inport
  State_iq_load_7_52d26 : Inport  Port=2
  State_iq_line_5_7_dcfea : Inport  Port=3
  State_iq_line_6_7_6dde0 : Inport  Port=4
  Add_13a66 : Sum
  Add_a4de4 : Sum
  Subtract_938a5 : Sum  Inputs=+-
  Blockout_iq_bus_7_06239 : Outport
  wires:
  Add_a4de4/1 -> Blockout_iq_bus_7_06239/1
  Subtract_938a5/1 -> Add_13a66/1
  Input_iq_GFL_DFIG_7_603eb/1 -> Subtract_938a5/1
  State_iq_load_7_52d26/1 -> Subtract_938a5/2
  Add_13a66/1 -> Add_a4de4/1
  State_iq_line_5_7_dcfea/1 -> Add_13a66/2
  State_iq_line_6_7_6dde0/1 -> Add_a4de4/2

== system IEEE30_case/AC_1/iq_bus_8_block ==
  note: iq_bus_8 in IEEE30_case
      | $\mathrm{iq}_{\mathrm{line},6,8}-\mathrm{iq}_{\mathrm{load},8}-\mathrm{iq}_{\mathrm{line},8,28}$
      | Automatically generated on 2025-11-01 18:42:48 .
  State_iq_load_8_74755 : Inport
  State_iq_line_6_8_44342 : Inport  Port=2
  State_iq_line_8_28_57c78 : Inport  Port=3
  Add_b2aaf : Sum
  Constant_-1_5eefb : Constant  Value=-1
  Product_343bf : Product
  Subtract_f050c : Sum  Inputs=+-
  Blockout_iq_bus_8_3c8c0 : Outport
  wires:
  State_iq_line_8_28_57c78/1 -> Subtract_f050c/2
  State_iq_line_6_8_44342/1 -> Add_b2aaf/2
  Product_343bf/1 -> Add_b2aaf/1
  Constant_-1_5eefb/1 -> Product_343bf/1
  State_iq_load_8_74755/1 -> Product_343bf/2
  Add_b2aaf/1 -> Subtract_f050c/1
  Subtract_f050c/1 -> Blockout_iq_bus_8_3c8c0/1

== system IEEE30_case/AC_1/iq_bus_9_block ==
  note: iq_bus_9 in IEEE30_case
      | $\mathrm{iq}_{\mathrm{line},6,9}-\mathrm{iq}_{\mathrm{line},9,10}-\mathrm{iq}_{\mathrm{line},9,11}$
      | Automatically generated on 2025-11-01 18:42:49 .
  State_iq_line_6_9_55e22 : Inport
  State_iq_line_9_10_59358 : Inport  Port=2
  State_iq_line_9_11_56031 : Inport  Port=3
  Subtract_2b03c : Sum  Inputs=+-
  Subtract_57f3b : Sum  Inputs=+-
  Blockout_iq_bus_9_1e267 : Outport
  wires:
  State_iq_line_6_9_55e22/1 -> Subtract_2b03c/1
  State_iq_line_9_11_56031/1 -> Subtract_57f3b/2
  Subtract_2b03c/1 -> Subtract_57f3b/1
  State_iq_line_9_10_59358/1 -> Subtract_2b03c/2
  Subtract_57f3b/1 -> Blockout_iq_bus_9_1e267/1

== system IEEE30_case/AC_1/vd_bus_13_out_block ==
  note: vd_bus_13_out in IEEE30_case
      | $\mathrm{vd}_{\mathrm{bus},13}$
      | Automatically generated on 2025-11-01 18:42:56 .
  State_vd_bus_13_f83b5 : Inport
  Blockout_vd_bus_13_out_de49d : Outport
  wires:
  State_vd_bus_13_f83b5/1 -> Blockout_vd_bus_13_out_de49d/1

== system IEEE30_case/AC_1/vd_bus_1_out_block ==
  note: vd_bus_1_out in IEEE30_case
      | $\mathrm{vd}_{\mathrm{bus},1}$
      | Automatically generated on 2025-11-01 18:42:32 .
  State_vd_bus_1_2d719 : Inport
  Blockout_vd_bus_1_out_a0239 : Outport
  wires:
  State_vd_bus_1_2d719/1 -> Blockout_vd_bus_1_out_a0239/1

== system IEEE30_case/AC_1/vd_bus_22_out_block ==
  note: vd_bus_22_out in IEEE30_case
      | $\mathrm{vd}_{\mathrm{bus},22}$
      | Automatically generated on 2025-11-01 18:43:12 .
  State_vd_bus_22_214cf : Inport
  Blockout_vd_bus_22_out_b1115 : Outport
  wires:
  State_vd_bus_22_214cf/1 -> Blockout_vd_bus_22_out_b1115/1

== system IEEE30_case/AC_1/vd_bus_23_out_block ==
  note: vd_bus_23_out in IEEE30_case
      | $\mathrm{vd}_{\mathrm{bus},23}$
      | Automatically generated on 2025-11-01 18:43:15 .
  State_vd_bus_23_a2fc7 : Inport
  Blockout_vd_bus_23_out_e84a6 : Outport
  wires:
  State_vd_bus_23_a2fc7/1 -> Blockout_vd_bus_23_out_e84a6/1

== system IEEE30_case/AC_1/vd_bus_27_out_block ==
  note: vd_bus_27_out in IEEE30_case
      | $\mathrm{vd}_{\mathrm{bus},27}$
      | Automatically generated on 2025-11-01 18:43:23 .
  State_vd_bus_27_9c8fe : Inport
  Blockout_vd_bus_27_out_73c03 : Outport
  wires:
  State_vd_bus_27_9c8fe/1 -> Blockout_vd_bus_27_out_73c03/1

== system IEEE30_case/AC_1/vd_bus_2_out_block ==
  note: vd_bus_2_out in IEEE30_case
      | $\mathrm{vd}_{\mathrm{bus},2}$
      | Automatically generated on 2025-11-01 18:42:34 .
  State_vd_bus_2_51c98 : Inport
  Blockout_vd_bus_2_out_6e542 : Outport
  wires:
  State_vd_bus_2_51c98/1 -> Blockout_vd_bus_2_out_6e542/1

== system IEEE30_case/AC_1/vd_bus_7_out_block ==
  note: vd_bus_7_out in IEEE30_case
      | $\mathrm{vd}_{\mathrm{bus},7}$
      | Automatically generated on 2025-11-01 18:42:44 .
  State_vd_bus_7_01f81 : Inport
  Blockout_vd_bus_7_out_4e91c : Outport
  wires:
  State_vd_bus_7_01f81/1 -> Blockout_vd_bus_7_out_4e91c/1

== system IEEE30_case/AC_1/vq_bus_13_out_block ==
  note: vq_bus_13_out in IEEE30_case
      | $\mathrm{vq}_{\mathrm{bus},13}$
      | Automatically generated on 2025-11-01 18:42:56 .
  State_vq_bus_13_2e03a : Inport
  Blockout_vq_bus_13_out_2bf25 : Outport
  wires:
  State_vq_bus_13_2e03a/1 -> Blockout_vq_bus_13_out_2bf25/1

== system IEEE30_case/AC_1/vq_bus_1_out_block ==
  note: vq_bus_1_out in IEEE30_case
      | $\mathrm{vq}_{\mathrm{bus},1}$
      | Automatically generated on 2025-11-01 18:42:32 .
  State_vq_bus_1_5ae62 : Inport
  Blockout_vq_bus_1_out_7cf09 : Outport
  wires:
  State_vq_bus_1_5ae62/1 -> Blockout_vq_bus_1_out_7cf09/1

== system IEEE30_case/AC_1/vq_bus_22_out_block ==
  note: vq_bus_22_out in IEEE30_case
      | $\mathrm{vq}_{\mathrm{bus},22}$
      | Automatically generated on 2025-11-01 18:43:13 .
  State_vq_bus_22_5efef : Inport
  Blockout_vq_bus_22_out_dafa4 : Outport
  wires:
  State_vq_bus_22_5efef/1 -> Blockout_vq_bus_22_out_dafa4/1

== system IEEE30_case/AC_1/vq_bus_23_out_block ==
  note: vq_bus_23_out in IEEE30_case
      | $\mathrm{vq}_{\mathrm{bus},23}$
      | Automatically generated on 2025-11-01 18:43:16 .
  State_vq_bus_23_75786 : Inport
  Blockout_vq_bus_23_out_e2230 : Outport
  wires:
  State_vq_bus_23_75786/1 -> Blockout_vq_bus_23_out_e2230/1

== system IEEE30_case/AC_1/vq_bus_27_out_block ==
  note: vq_bus_27_out in IEEE30_case
      | $\mathrm{vq}_{\mathrm{bus},27}$
      | Automatically generated on 2025-11-01 18:43:23 .
  State_vq_bus_27_50cd3 : Inport
  Blockout_vq_bus_27_out_7c7b9 : Outport
  wires:
  State_vq_bus_27_50cd3/1 -> Blockout_vq_bus_27_out_7c7b9/1

== system IEEE30_case/AC_1/vq_bus_2_out_block ==
  note: vq_bus_2_out in IEEE30_case
      | $\mathrm{vq}_{\mathrm{bus},2}$
      | Automatically generated on 2025-11-01 18:42:35 .
  State_vq_bus_2_331ca : Inport
  Blockout_vq_bus_2_out_9085b : Outport
  wires:
  State_vq_bus_2_331ca/1 -> Blockout_vq_bus_2_out_9085b/1

== system IEEE30_case/AC_1/vq_bus_7_out_block ==
  note: vq_bus_7_out in IEEE30_case
      | $\mathrm{vq}_{\mathrm{bus},7}$
      | Automatically generated on 2025-11-01 18:42:45 .
  State_vq_bus_7_4fcda : Inport
  Blockout_vq_bus_7_out_1686e : Outport
  wires:
  State_vq_bus_7_4fcda/1 -> Blockout_vq_bus_7_out_1686e/1

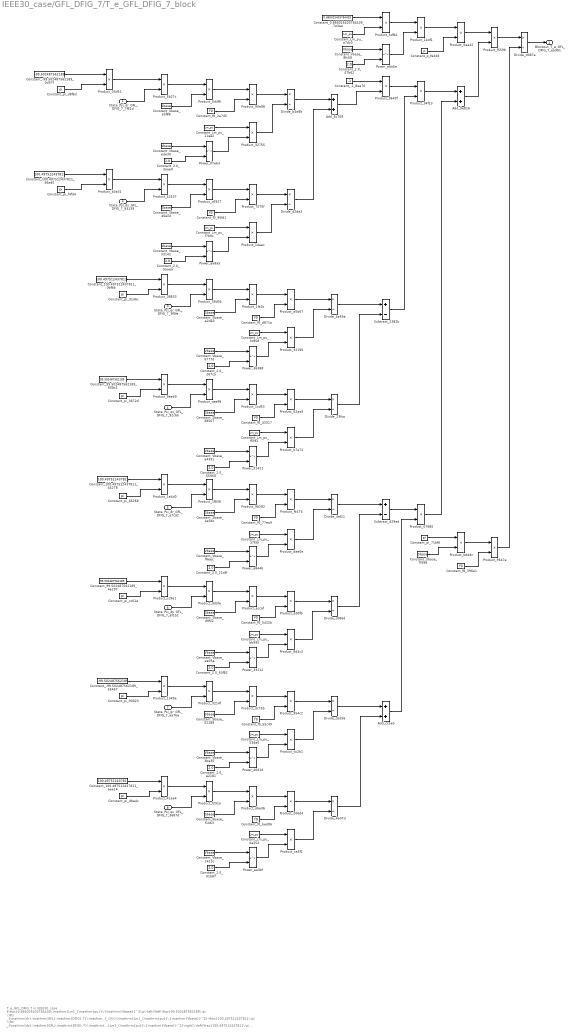
== system IEEE30_case/GFL_DFIG_7/T_e_GFL_DFIG_7_block ==
  note: T_e_GFL_DFIG_7 in IEEE30_case
      | $\frac{0.866025403784439\,\mathrm{Lm}_{\mathrm{pu}}\,{\mathrm{Vbase}}^2\,p\,\left(\left(\frac{99.502487562189\,\pi \,\Psi _{\mathrm{dr},\mathrm{GFL},\mathrm{DFIG},7}\,\mathrm{Sbase}\,f_{0}}{\mathrm{Lm}_{\mathrm{pu}}\,{\mathrm{Vbase}}^2}-\frac{100.497512437811\,\pi \,\Psi _{\mathrm{ds},\mathrm{GFL},\mathrm{DFIG},7}\,\mathrm{Sbase}\,f_{0}}{\mathrm{Lm}_{\mathrm{pu}}\,{\mathrm{Vbase}}^2}\right)\,\left(\frac{100.497512437811\,\pi \,\Psi _{\mathrm{qr},\mathrm{GFL},\mathrm{DFIG},7}\,\mathrm{Sbase}\,f_{0}}{\mathrm{Lm}_{\mathrm{pu}}\,{\mathrm{Vbase}}^2}-\frac{99.502487562189\,\pi \,\Psi _{\mathrm{qs},\mathrm{GFL},\mathrm{DFIG},7}\,\mathrm{Sbase}\,f_{0}}{\mathrm{Lm}_{\mathrm{pu}}\,{\mathrm{Vbase}}^2}\right)-\left(\frac{100.497512437811\,\pi \,\Psi _{\mathrm{dr},\mathrm{GFL},\mathrm{DFIG},7}\,\mathrm{Sbase}\,f_{0}}{\mathrm{Lm}_{\mathrm{pu}}\,{\mathrm{Vbase}}^2}-\frac{99.502487562189\,\pi \,\Psi _{\mathrm{ds},\mathrm{GFL},\mathrm{DFIG},7}\,\mathrm{Sbase}\,f_{0}}{\mathrm{Lm}_{\mathrm{pu}}\,{\mathrm{Vbase}}^2}\right)\,\left(\frac{99.502487562189\,\pi \,\Psi _{\mathrm{qr},\mathrm{GFL},\mathrm{DFIG},7}\,\mathrm{Sbase}\,f_{0}}{\mathrm{Lm}_{\mathrm{pu}}\,{\mathrm{Vbase}}^2}-\frac{100.497512437811\,\pi \,\Psi _{\mathrm{qs},\mathrm{GFL},\mathrm{DFIG},7}\,\mathrm{Sbase}\,f_{0}}{\mathrm{Lm}_{\mathrm{pu}}\,{\mathrm{Vbase}}^2}\right)\right)}{\mathrm{Sbase}\,f_{0}\,\pi }$
      | Automatically generated on 2025-11-01 18:34:27 .
  State_Psi_dr_GFL_DFIG_7_7f61d : Inport
  State_Psi_ds_GFL_DFIG_7_93139 : Inport  Port=2
  State_Psi_qr_GFL_DFIG_7_3f5fe : Inport  Port=3
  State_Psi_qs_GFL_DFIG_7_92c6b : Inport  Port=4
  State_Psi_dr_GFL_DFIG_7_e7cd2 : Inport  Port=5
  State_Psi_ds_GFL_DFIG_7_ef1b2 : Inport  Port=6
  State_Psi_qr_GFL_DFIG_7_aa7be : Inport  Port=7
  State_Psi_qs_GFL_DFIG_7_3687d : Inport  Port=8
  Add_6c769 : Sum
  Add_9e816 : Sum
  Add_ccaab : Sum
  Constant_-1_8ea76 : Constant  Value=-1
  Constant_-99.502487562189_0d37f : Constant  Value=-99.502487562189
  Constant_-99.502487562189_55457 : Constant  Value=-99.502487562189
  Constant_0.866025403784439_7e3ee : Constant  Value=0.866025403784439
  Constant_100.497512437811_0bfbb : Constant  Value=100.497512437811
  Constant_100.497512437811_36ad0 : Constant  Value=100.497512437811
  Constant_100.497512437811_44278 : Constant  Value=100.497512437811
  Constant_100.497512437811_aee14 : Constant  Value=100.497512437811
  Constant_2.0_01b87 : Constant  Value=2.0
  Constant_2.0_21c8f : Constant  Value=2.0
  Constant_2.0_267ca : Constant  Value=2.0
  Constant_2.0_3aae9 : Constant  Value=2.0
  Constant_2.0_47b62 : Constant  Value=2.0
  Constant_2.0_55950 : Constant  Value=2.0
  Constant_2.0_5aaea : Constant  Value=2.0
  Constant_2.0_63f82 : Constant  Value=2.0
  Constant_2.0_a2181 : Constant  Value=2.0
  Constant_99.502487562189_4e297 : Constant  Value=99.502487562189
  Constant_99.502487562189_608c1 : Constant  Value=99.502487562189
  Constant_Lm_pu_0a254 : Constant  Value=Lm_pu
  Constant_Lm_pu_11ee2 : Constant  Value=Lm_pu
  Constant_Lm_pu_37f39 : Constant  Value=Lm_pu
  Constant_Lm_pu_3c958 : Constant  Value=Lm_pu
  Constant_Lm_pu_53da0 : Constant  Value=Lm_pu
  Constant_Lm_pu_a7dc0 : Constant  Value=Lm_pu
  Constant_Lm_pu_bb995 : Constant  Value=Lm_pu
  Constant_Lm_pu_f7b0c : Constant  Value=Lm_pu
  Constant_Lm_pu_ff292 : Constant  Value=Lm_pu
  Constant_Sbase_02188 : Constant  Value=Sbase
  Constant_Sbase_38567 : Constant  Value=Sbase
  Constant_Sbase_46ecd : Constant  Value=Sbase
  Constant_Sbase_4e3bc : Constant  Value=Sbase
  Constant_Sbase_7f398 : Constant  Value=Sbase
  Constant_Sbase_a2da3 : Constant  Value=Sbase
  Constant_Sbase_abf88 : Constant  Value=Sbase
  Constant_Sbase_d9fc2 : Constant  Value=Sbase
  Constant_Sbase_f1063 : Constant  Value=Sbase
  Constant_Vbase_2413c : Constant  Value=Vbase
  Constant_Vbase_33142 : Constant  Value=Vbase
  Constant_Vbase_3be35 : Constant  Value=Vbase
  Constant_Vbase_6777d : Constant  Value=Vbase
  Constant_Vbase_8fc58 : Constant  Value=Vbase
  Constant_Vbase_a4391 : Constant  Value=Vbase
  Constant_Vbase_ea05a : Constant  Value=Vbase
  Constant_Vbase_ede30 : Constant  Value=Vbase
  Constant_Vbase_f8eec : Constant  Value=Vbase
  Constant_f0_2a745 : Constant  Value=f0
  Constant_f0_396e1 : Constant  Value=f0
  Constant_f0_43317 : Constant  Value=f0
  Constant_f0_5432b : Constant  Value=f0
  Constant_f0_55c49 : Constant  Value=f0
  Constant_f0_77ea9 : Constant  Value=f0
  Constant_f0_95fd1 : Constant  Value=f0
  Constant_f0_bed96 : Constant  Value=f0
  Constant_f0_d871a : Constant  Value=f0
  Constant_p_fe43d : Constant  Value=p
  Constant_pi_31d6c : Constant  Value=pi
  Constant_pi_3672d : Constant  Value=pi
  Constant_pi_66268 : Constant  Value=pi
  Constant_pi_71bf8 : Constant  Value=pi
  Constant_pi_90020 : Constant  Value=pi
  Constant_pi_cc01e : Constant  Value=pi
  Constant_pi_d8f6d : Constant  Value=pi
  Constant_pi_dba4c : Constant  Value=pi
  Constant_pi_f4fd4 : Constant  Value=pi
  Divide_23fca : Product  Inputs=*/
  Divide_4e07d : Product  Inputs=*/
  Divide_4e59a : Product  Inputs=*/
  Divide_4ef11 : Product  Inputs=*/
  Divide_b4a8b : Product  Inputs=*/
  Divide_c086d : Product  Inputs=*/
  Divide_cbd56 : Product  Inputs=*/
  Divide_d087a : Product  Inputs=*/
  Divide_d2de3 : Product  Inputs=*/
  Power_07e63 : Math  Operator=pow
  Power_31421 : Math  Operator=pow
  Power_33212 : Math  Operator=pow
  Power_36388 : Math  Operator=pow
  Power_40d1d : Math  Operator=pow
  Power_a844b : Math  Operator=pow
  Power_aa3bf : Math  Operator=pow
  Power_aa8a5 : Math  Operator=pow
  Power_e6a5e : Math  Operator=pow
  Product_03d51 : Product
  Product_07680 : Product
  Product_08833 : Product
  Product_0aa42 : Product
  Product_1349e : Product
  Product_14df1 : Product
  Product_14eec : Product
  Product_1cd53 : Product
  Product_1e4d0 : Product
  Product_1f836 : Product
  Product_1fa3c : Product
  Product_206d4 : Product
  Product_3214f : Product
  Product_32190 : Product
  Product_32755 : Product
  Product_34f13 : Product
  Product_39d04 : Product
  Product_41ea4 : Product
  Product_42537 : Product
  Product_5b27c : Product
  Product_5d4f6 : Product
  Product_5dfb1 : Product
  Product_62aa9 : Product
  Product_7075f : Product
  Product_8d3c3 : Product
  Product_90e98 : Product
  Product_9547e : Product
  Product_954c2 : Product
  Product_9649f : Product
  Product_9b282 : Product
  Product_9ee49 : Product
  Product_a5b67 : Product
  Product_a99fb : Product
  Product_b3a31 : Product
  Product_b7a72 : Product
  Product_bdddc : Product
  Product_c6927 : Product
  Product_ca5f2 : Product
  Product_cc2b1 : Product
  Product_cc9e1 : Product
  Product_cee98 : Product
  Product_dae0e : Product
  Product_dbe36 : Product
  Product_dc75b : Product
  Product_dd5fe : Product
  Product_eccaf : Product
  Product_f291a : Product
  Product_f559b : Product
  Product_fb174 : Product
  Subtract_2382b : Sum  Inputs=+-
  Subtract_d29ed : Sum  Inputs=+-
  Blockout_T_e_GFL_DFIG_7_ea981 : Outport
  wires:
  Divide_4ef11/1 -> Subtract_d29ed/1
  State_Psi_qr_GFL_DFIG_7_3f5fe/1 -> Product_39d04/2
  Constant_-99.502487562189_0d37f/1 -> Product_03d51/1
  Constant_pi_d8f6d/1 -> Product_03d51/2
  Constant_f0_95fd1/1 -> Product_7075f/2
  Product_62aa9/1 -> Divide_23fca/1
  State_Psi_ds_GFL_DFIG_7_ef1b2/1 -> Product_dd5fe/2
  State_Psi_ds_GFL_DFIG_7_93139/1 -> Product_42537/2
  Constant_99.502487562189_4e297/1 -> Product_cc9e1/1
  Constant_100.497512437811_36ad0/1 -> Product_b3a31/1
  Constant_Lm_pu_11ee2/1 -> Product_32755/1
  Constant_Lm_pu_a7dc0/1 -> Product_5dfb1/2
  State_Psi_dr_GFL_DFIG_7_7f61d/1 -> Product_5b27c/2
  State_Psi_qs_GFL_DFIG_7_3687d/1 -> Product_f291a/2
  Product_41ea4/1 -> Product_f291a/1
  Constant_pi_cc01e/1 -> Product_cc9e1/2
  Product_9ee49/1 -> Product_cee98/1
  Constant_pi_f4fd4/1 -> Product_b3a31/2
  Product_03d51/1 -> Product_5b27c/1
  State_Psi_qs_GFL_DFIG_7_92c6b/1 -> Product_cee98/2
  Product_cc9e1/1 -> Product_dd5fe/1
  Constant_100.497512437811_aee14/1 -> Product_41ea4/1
  Constant_99.502487562189_608c1/1 -> Product_9ee49/1
  Product_b3a31/1 -> Product_42537/1
  Constant_Sbase_abf88/1 -> Product_5d4f6/2
  Product_1e4d0/1 -> Product_1f836/1
  Constant_-99.502487562189_55457/1 -> Product_1349e/1
  Constant_100.497512437811_0bfbb/1 -> Product_08833/1
  Constant_pi_31d6c/1 -> Product_08833/2
  Product_1f836/1 -> Product_9b282/1
  Divide_b4a8b/1 -> Add_6c769/1
  Constant_pi_3672d/1 -> Product_9ee49/2
  Product_dd5fe/1 -> Product_eccaf/1
  Product_42537/1 -> Product_c6927/1
  Constant_100.497512437811_44278/1 -> Product_1e4d0/1
  State_Psi_qr_GFL_DFIG_7_aa7be/1 -> Product_3214f/2
  Divide_4e59a/1 -> Subtract_2382b/1
  Constant_pi_66268/1 -> Product_1e4d0/2
  Product_39d04/1 -> Product_1fa3c/1
  Constant_pi_90020/1 -> Product_1349e/2
  Power_e6a5e/1 -> Product_14df1/2
  Product_cee98/1 -> Product_1cd53/1
  Constant_pi_dba4c/1 -> Product_41ea4/2
  Product_5b27c/1 -> Product_5d4f6/1
  Constant_Vbase_f8eec/1 -> Power_a844b/1
  Constant_2.0_267ca/1 -> Power_36388/2
  Constant_Vbase_ede30/1 -> Power_07e63/1
  Constant_2.0_21c8f/1 -> Power_a844b/2
  Constant_2.0_3aae9/1 -> Power_07e63/2
  Constant_Sbase_d9fc2/1 -> Product_eccaf/2
  Product_dbe36/1 -> Product_206d4/1
  Constant_Sbase_46ecd/1 -> Product_c6927/2
  Constant_Vbase_ea05a/1 -> Power_33212/1
  Constant_2.0_55950/1 -> Power_31421/2
  Constant_Vbase_33142/1 -> Power_aa8a5/1
  Constant_2.0_63f82/1 -> Power_33212/2
  Constant_2.0_5aaea/1 -> Power_aa8a5/2
  Product_1349e/1 -> Product_3214f/1
  Product_08833/1 -> Product_39d04/1
  Product_a5b67/1 -> Divide_4e59a/1
  State_Psi_dr_GFL_DFIG_7_e7cd2/1 -> Product_1f836/2
  Constant_Vbase_6777d/1 -> Power_36388/1
  Product_5d4f6/1 -> Product_90e98/1
  Constant_f0_2a745/1 -> Product_90e98/2
  Power_07e63/1 -> Product_32755/2
  Constant_f0_bed96/1 -> Product_206d4/2
  Product_c6927/1 -> Product_7075f/1
  Constant_Lm_pu_f7b0c/1 -> Product_14eec/1
  Power_aa8a5/1 -> Product_14eec/2
  Constant_Sbase_a2da3/1 -> Product_1fa3c/2
  Constant_Sbase_38567/1 -> Product_1cd53/2
  Constant_Vbase_a4391/1 -> Power_31421/1
  Constant_Sbase_4e3bc/1 -> Product_9b282/2
  Product_3214f/1 -> Product_dc75b/1
  Constant_Sbase_02188/1 -> Product_dc75b/2
  Constant_Vbase_3be35/1 -> Power_40d1d/1
  Constant_2.0_a2181/1 -> Power_40d1d/2
  Product_f291a/1 -> Product_dbe36/1
  Product_7075f/1 -> Divide_d2de3/1
  Constant_Sbase_f1063/1 -> Product_dbe36/2
  Constant_Vbase_2413c/1 -> Power_aa3bf/1
  Constant_2.0_01b87/1 -> Power_aa3bf/2
  Divide_c086d/1 -> Subtract_d29ed/2
  Product_90e98/1 -> Divide_b4a8b/1
  Product_32755/1 -> Divide_b4a8b/2
  Product_14eec/1 -> Divide_d2de3/2
  Product_1fa3c/1 -> Product_a5b67/1
  Constant_f0_d871a/1 -> Product_a5b67/2
  Constant_Lm_pu_3c958/1 -> Product_32190/1
  Constant_-1_8ea76/1 -> Product_9649f/1
  Power_36388/1 -> Product_32190/2
  Constant_pi_71bf8/1 -> Product_bdddc/1
  Product_1cd53/1 -> Product_62aa9/1
  Constant_f0_43317/1 -> Product_62aa9/2
  Constant_Lm_pu_ff292/1 -> Product_b7a72/1
  Power_31421/1 -> Product_b7a72/2
  Constant_Sbase_7f398/1 -> Product_bdddc/2
  Product_9b282/1 -> Product_fb174/1
  Constant_f0_77ea9/1 -> Product_fb174/2
  Constant_Lm_pu_37f39/1 -> Product_dae0e/1
  Power_a844b/1 -> Product_dae0e/2
  Product_eccaf/1 -> Product_a99fb/1
  Constant_f0_5432b/1 -> Product_a99fb/2
  Constant_Lm_pu_bb995/1 -> Product_8d3c3/1
  Power_33212/1 -> Product_8d3c3/2
  Product_dc75b/1 -> Product_954c2/1
  Constant_f0_55c49/1 -> Product_954c2/2
  Constant_Lm_pu_53da0/1 -> Product_cc2b1/1
  Power_40d1d/1 -> Product_cc2b1/2
  Constant_Lm_pu_0a254/1 -> Product_ca5f2/1
  Power_aa3bf/1 -> Product_ca5f2/2
  Divide_d2de3/1 -> Add_6c769/2
  Product_32190/1 -> Divide_4e59a/2
  Product_b7a72/1 -> Divide_23fca/2
  Product_fb174/1 -> Divide_4ef11/1
  Product_dae0e/1 -> Divide_4ef11/2
  Product_a99fb/1 -> Divide_c086d/1
  Product_8d3c3/1 -> Divide_c086d/2
  Product_954c2/1 -> Divide_cbd56/1
  Product_cc2b1/1 -> Divide_cbd56/2
  Product_206d4/1 -> Divide_4e07d/1
  Product_ca5f2/1 -> Divide_4e07d/2
  Constant_0.866025403784439_7e3ee/1 -> Product_5dfb1/1
  Constant_Vbase_8fc58/1 -> Power_e6a5e/1
  Constant_2.0_47b62/1 -> Power_e6a5e/2
  Add_6c769/1 -> Product_9649f/2
  Divide_23fca/1 -> Subtract_2382b/2
  Divide_cbd56/1 -> Add_ccaab/1
  Divide_4e07d/1 -> Add_ccaab/2
  Product_5dfb1/1 -> Product_14df1/1
  Product_9649f/1 -> Product_34f13/1
  Subtract_2382b/1 -> Product_34f13/2
  Subtract_d29ed/1 -> Product_07680/1
  Add_ccaab/1 -> Product_07680/2
  Product_14df1/1 -> Product_0aa42/1
  Constant_p_fe43d/1 -> Product_0aa42/2
  Product_34f13/1 -> Add_9e816/1
  Product_07680/1 -> Add_9e816/2
  Product_0aa42/1 -> Product_f559b/1
  Add_9e816/1 -> Product_f559b/2
  Product_bdddc/1 -> Product_9547e/1
  Constant_f0_396e1/1 -> Product_9547e/2
  Product_f559b/1 -> Divide_d087a/1
  Product_9547e/1 -> Divide_d087a/2
  Divide_d087a/1 -> Blockout_T_e_GFL_DFIG_7_ea981/1

== system IEEE30_case/GFL_DFIG_7/d_Phi_ga_GFL_DFIG_7_block ==
  note: d_Phi_ga_GFL_DFIG_7 in IEEE30_case
      | $4\,\mathrm{Lg}\,{f_{0}}^2\,\pi ^2\,\left(\mathrm{Igq}_{\mathrm{ref}}-i_{\mathrm{gq},\mathrm{GFL},\mathrm{DFIG},7}\right)$
      | Automatically generated on 2025-11-01 18:34:02 .
  State_i_gq_GFL_DFIG_7_ca300 : Inport
  Constant_2.0_c0566 : Constant  Value=2.0
  Constant_2.0_d6eb3 : Constant  Value=2.0
  Constant_4.0_1ae90 : Constant  Value=4.0
  Constant_Igq_ref_22f44 : Constant  Value=Igq_ref
  Constant_Lg_5a077 : Constant  Value=Lg
  Constant_f0_66864 : Constant  Value=f0
  Constant_pi_c92a6 : Constant  Value=pi
  Power_24233 : Math  Operator=pow
  Power_9bf06 : Math  Operator=pow
  Product_a2166 : Product
  Product_cf70e : Product
  Product_e1e04 : Product
  Product_edec9 : Product
  Subtract_1472e : Sum  Inputs=+-
  Blockout_d_Phi_ga_GFL_DFIG_7_179fc : Outport
  wires:
  Constant_f0_66864/1 -> Power_9bf06/1
  Constant_pi_c92a6/1 -> Power_24233/1
  Constant_2.0_d6eb3/1 -> Power_24233/2
  Constant_4.0_1ae90/1 -> Product_a2166/1
  Subtract_1472e/1 -> Product_cf70e/2
  Constant_Lg_5a077/1 -> Product_e1e04/2
  Product_a2166/1 -> Product_e1e04/1
  State_i_gq_GFL_DFIG_7_ca300/1 -> Subtract_1472e/2
  Power_24233/1 -> Product_a2166/2
  Constant_2.0_c0566/1 -> Power_9bf06/2
  Product_e1e04/1 -> Product_edec9/1
  Power_9bf06/1 -> Product_edec9/2
  Constant_Igq_ref_22f44/1 -> Subtract_1472e/1
  Product_edec9/1 -> Product_cf70e/1
  Product_cf70e/1 -> Blockout_d_Phi_ga_GFL_DFIG_7_179fc/1
